simulink model "ScaraRobotApresentacao2023"  (R2024a)
settings: Solver=VariableStepAuto  StartTime=0.0  StopTime=200  RelTol=1e-3
model workspace: external: MATLAB File C:\Users\lucas\OneDrive\Documents\MATLAB\Robotica_2023b\ScaraRobot_DataFile.m (data not in the file)
values from neighbouring files (symbols this model uses):
  I = cell(1,n)    [calcularDinamica.m]    (also in inicializacaoAntropomorfico.m = {I1, I2, I3, I4, I5, I6, I7})
  L = [L1, L2, L3, L4, L5, L6, L7]    [inicializacaoAntropomorfico.m]
  Lcm = {Lcm1, Lcm2, Lcm3, Lcm4, Lcm5, Lcm6, Lcm7}    [inicializacaoAntropomorfico.m]
  m = [m1, m2, m3, m4, m5, m6, m7]    [inicializacaoAntropomorfico.m]
  Pf = [  0.05    [inicializacaoAntropomorfico.m]
  Pi = [  0.2    [inicializacaoAntropomorfico.m]
  Raio = [0]    [inicializacaoAntropomorfico.m]
  Sentido = [0]    [inicializacaoAntropomorfico.m]
  Tipo = [1]    [inicializacaoAntropomorfico.m]
undefined symbols (not defined in the file or in its folder): Lx1, Lx2, smiData, X, Y, Z
libraries: sm_lib x25, nesl_utility x5
(part 4 of 10)

== matlab function ScaraRobotApresentacao2023/Dinamica/MATLAB Function2 ==
  data: G output; I parameter; L parameter; Lcm parameter; Q input
function G = func_G(I, L, Lcm, Q)
%func_G
%    OUT1 = func_G(Lx2,Lx3,Lxcm2,Lxcm3,Lxcm4,Lxcm5,Lxcm6,Lycm4,Lycm5,Lycm6,Lz4,Lz5,Lzcm2,Lzcm3,Lzcm4,Lzcm5,Lzcm6,Q2,Q3,Q4,Q5,Q6,G2,G3,G4,G5,G6,M2,M3,M4,M5,M6)

%    This function was generated by the Symbolic Math Toolbox version 24.1.
%    30-Apr-2025 06:22:17

Q1  = Q(1);
Q2  = Q(2);
Q3  = Q(3);
Q4  = Q(4);
Q5  = Q(5);
Q6  = Q(6);

Lx1 = L{1}(1);
Ly1 = L{1}(2);
Lz1 = L{1}(3);

Lx2 = L{2}(1);
Ly2 = L{2}(2);
Lz2 = L{2}(3);

Lx3 = L{3}(1);
Ly3 = L{3}(2);
Lz3 = L{3}(3);

Lx4 = L{4}(1);
Ly4 = L{4}(2);
Lz4 = L{4}(3);

Lx5 = L{5}(1);
Ly5 = L{5}(2);
Lz5 = L{5}(3);

Lx6 = L{6}(1);
Ly6 = L{6}(2);
Lz6 = L{6}(3);

Lxcm1 = Lcm{1}(1);
Lycm1 = Lcm{1}(2);
Lzcm1 = Lcm{1}(3);

Lxcm2 = Lcm{2}(1);
Lycm2 = Lcm{2}(2);
Lzcm2 = Lcm{2}(3);

Lxcm3 = Lcm{3}(1);
Lycm3 = Lcm{3}(2);
Lzcm3 = Lcm{3}(3);

Lxcm4 = Lcm{4}(1);
Lycm4 = Lcm{4}(2);
Lzcm4 = Lcm{4}(3);

Lxcm5 = Lcm{5}(1);
Lycm5 = Lcm{5}(2);
Lzcm5 = Lcm{5}(3);

Lxcm6 = Lcm{6}(1);
Lycm6 = Lcm{6}(2);
Lzcm6 = Lcm{6}(3);

Ixx1 = I{1}(1,1);
Ixy1 = I{1}(1,2);
Ixz1 = I{1}(1,3);
Iyx1 = I{1}(2,1);
Iyy1 = I{1}(2,2);
Iyz1 = I{1}(2,3);
Izx1 = I{1}(3,1);
Izy1 = I{1}(3,2);
Izz1 = I{1}(3,3);

Ixx2 = I{2}(1,1);
Ixy2 = I{2}(1,2);
Ixz2 = I{2}(1,3);
Iyx2 = I{2}(2,1);
Iyy2 = I{2}(2,2);
Iyz2 = I{2}(2,3);
Izx2 = I{2}(3,1);
Izy2 = I{2}(3,2);
Izz2 = I{2}(3,3);

Ixx3 = I{3}(1,1);
Ixy3 = I{3}(1,2);
Ixz3 = I{3}(1,3);
Iyx3 = I{3}(2,1);
Iyy3 = I{3}(2,2);
Iyz3 = I{3}(2,3);
Izx3 = I{3}(3,1);
Izy3 = I{3}(3,2);
Izz3 = I{3}(3,3);

Ixx4 = I{4}(1,1);
Ixy4 = I{4}(1,2);
Ixz4 = I{4}(1,3);
Iyx4 = I{4}(2,1);
Iyy4 = I{4}(2,2);
Iyz4 = I{4}(2,3);
Izx4 = I{4}(3,1);
Izy4 = I{4}(3,2);
Izz4 = I{4}(3,3);

Ixx5 = I{5}(1,1);
Ixy5 = I{5}(1,2);
Ixz5 = I{5}(1,3);
Iyx5 = I{5}(2,1);
Iyy5 = I{5}(2,2);
Iyz5 = I{5}(2,3);
Izx5 = I{5}(3,1);
Izy5 = I{5}(3,2);
Izz5 = I{5}(3,3);

Ixx6 = I{6}(1,1);
Ixy6 = I{6}(1,2);
Ixz6 = I{6}(1,3);
Iyx6 = I{6}(2,1);
Iyy6 = I{6}(2,2);
Iyz6 = I{6}(2,3);
Izx6 = I{6}(3,1);
Izy6 = I{6}(3,2);
Izz6 = I{6}(3,3);

t2 = cos(Q2);
t3 = cos(Q3);
t4 = cos(Q4);
t5 = cos(Q5);
t6 = cos(Q6);
t7 = sin(Q2);
t8 = sin(Q3);
t9 = sin(Q4);
t10 = sin(Q5);
t11 = sin(Q6);
t12 = Q2+Q3;
t13 = cos(t12);
t14 = sin(t12);
t15 = t2.*t3;
t16 = t7.*t8;
t17 = -t16;
t18 = t15+t17;
t19 = Lx3.*t18;
et1 = -Lx2.*g3.*m3.*t2-Lx2.*g4.*m4.*t2-Lx2.*g5.*m5.*t2-Lx2.*g6.*m6.*t2-Lx3.*g4.*m4.*t15+Lx3.*g4.*m4.*t16-Lx3.*g5.*m5.*t15-Lx3.*g6.*m6.*t13+Lx3.*g5.*m5.*t16-Lxcm2.*g2.*m2.*t2-Lxcm3.*g3.*m3.*t13-Lz4.*g6.*m6.*t14-Lzcm2.*g2.*m2.*t7-Lzcm3.*g3.*m3.*t14-Lzcm4.*g4.*m4.*t14-Lxcm4.*g4.*m4.*t4.*t13+Lxcm5.*g5.*m5.*t10.*t14+Lycm4.*g4.*m4.*t9.*t13+Lycm5.*g5.*m5.*t9.*t13-Lz4.*g5.*m5.*t2.*t8-Lz4.*g5.*m5.*t3.*t7-Lz5.*g6.*m6.*t5.*t14-Lzcm5.*g5.*m5.*t5.*t14-Lzcm6.*g6.*m6.*t5.*t14-Lxcm5.*g5.*m5.*t4.*t5.*t13+Lxcm6.*g6.*m6.*t6.*t10.*t14+Lxcm6.*g6.*m6.*t9.*t11.*t13+Lycm6.*g6.*m6.*t6.*t9.*t13;
et2 = -Lycm6.*g6.*m6.*t10.*t11.*t14-Lz5.*g6.*m6.*t4.*t10.*t13-Lzcm5.*g5.*m5.*t4.*t10.*t13-Lzcm6.*g6.*m6.*t4.*t10.*t13-Lxcm6.*g6.*m6.*t4.*t5.*t6.*t13+Lycm6.*g6.*m6.*t4.*t5.*t11.*t13;
mt1 = [0.0;et1+et2;-g6.*m6.*(Lx3.*t13+Lz4.*t14+Lz5.*t5.*t14+Lzcm6.*t5.*t14-Lxcm6.*t6.*t10.*t14-Lxcm6.*t9.*t11.*t13-Lycm6.*t6.*t9.*t13+Lycm6.*t10.*t11.*t14+Lz5.*t4.*t10.*t13+Lzcm6.*t4.*t10.*t13+Lxcm6.*t4.*t5.*t6.*t13-Lycm6.*t4.*t5.*t11.*t13)-g4.*m4.*(t19+Lzcm4.*t14+Lxcm4.*t4.*t13-Lycm4.*t9.*t13)-g5.*m5.*(t19-Lxcm5.*(t10.*t14-t4.*t5.*t13)+Lzcm5.*(t5.*t14+t4.*t10.*t13)+Lz4.*(t2.*t8+t3.*t7)-Lycm5.*t9.*t13)-g3.*m3.*(Lxcm3.*t13+Lzcm3.*t14)];
mt2 = [t14.*(Lxcm4.*g4.*m4.*t9+Lycm4.*g4.*m4.*t4+Lycm5.*g5.*m5.*t4+Lxcm5.*g5.*m5.*t5.*t9+Lxcm6.*g6.*m6.*t4.*t11+Lycm6.*g6.*m6.*t4.*t6+Lz5.*g6.*m6.*t9.*t10+Lzcm5.*g5.*m5.*t9.*t10+Lzcm6.*g6.*m6.*t9.*t10+Lxcm6.*g6.*m6.*t5.*t6.*t9-Lycm6.*g6.*m6.*t5.*t9.*t11);-g5.*m5.*(Lxcm5.*(t5.*t13-t4.*t10.*t14)+Lzcm5.*(t10.*t13+t4.*t5.*t14))-g6.*m6.*(Lz5.*t10.*t13+Lzcm6.*t10.*t13+Lxcm6.*t5.*t6.*t13-Lycm6.*t5.*t11.*t13+Lz5.*t4.*t5.*t14+Lzcm6.*t4.*t5.*t14-Lxcm6.*t4.*t6.*t10.*t14+Lycm6.*t4.*t10.*t11.*t14);g6.*m6.*(Lxcm6.*t6.*t9.*t14+Lxcm6.*t10.*t11.*t13+Lycm6.*t6.*t10.*t13-Lycm6.*t9.*t11.*t14+Lxcm6.*t4.*t5.*t11.*t14+Lycm6.*t4.*t5.*t6.*t14)];
G = [mt1;mt2];
end
